simulink model "DCMotorModel"  (R2025a)
settings: Solver=VariableStepAuto  StartTime=0.0  StopTime=10.0  RelTol=1e-3
undefined symbols (not defined in the file): den_armature, den_load, Kb, Kma, num_armature, num_load, Tl, Va
settings Model: Creator=CHIBIK  LastModifiedBy=CHIBIK
settings RTWCC: GPUComputeCapability=3.5

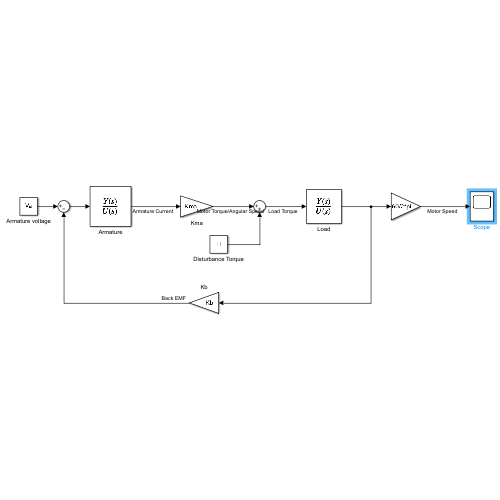
[thumbnail: Simulink's stored preview of the top-level diagram]
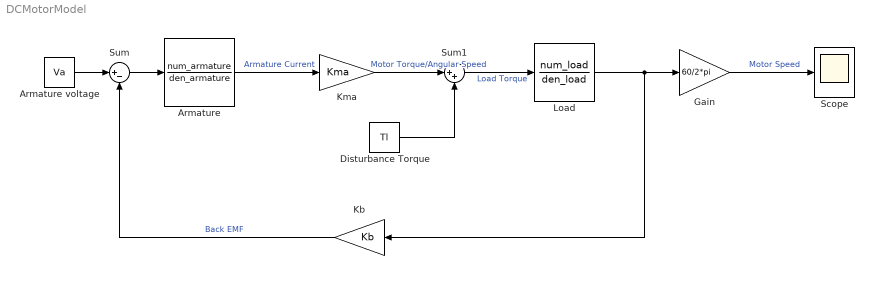
== system DCMotorModel ==
  Armature : TransferFcn  Numerator=num_armature  Denominator=den_armature
  Armature voltage : Constant  Value=Va
  Disturbance Torque : Constant  Value=Tl
  Gain : Gain  Gain=60/2*pi
  Kb : Gain  Gain=Kb
  Kma : Gain  Gain=Kma
  Load : TransferFcn  Numerator=num_load  Denominator=den_load
  Scope : Scope
      settings: Title=Motor Speed against Time  ActiveDisplayYMinimum=0  ActiveDisplayYMaximum=60099.445794274929  DataLoggingVariableName=MotorSpeed_data
  Sum : Sum  Inputs=|+-
  Sum1 : Sum  Inputs=|++
  wires:
  Armature voltage/1 -> Sum/1
  Sum/1 -> Armature/1
  Armature/1 -> Kma/1  "Armature Current"
  Kma/1 -> Sum1/1  "Motor Torque/Angular Speed"
  Sum1/1 -> Load/1  "Load Torque"
  Disturbance Torque/1 -> Sum1/2
  Load/1 -> Kb/1, Gain/1
  Kb/1 -> Sum/2  "Back EMF"
  Gain/1 -> Scope/1  "Motor Speed"
